simulink model "DroopGFM_sps"  (R2024b)
settings: Solver=ode3  StartTime=0.0  StopTime=10  FixedStep=5e-6  RelTol=1e-3
InitFcn:
  | fsw=10e3;
  | %Ts=1/(fsw*50); %1e-6
  | Ts=1/(fsw*20);  %5e-6
  | 
  | Vodref= 480*sqrt(2/3);
  | Vdc=1000;
  | w0=2*pi*60;
  | 
  | Lf=3.5e-3;
  | Rf=0.1;
  | Cf=50e-6;
  | Lc=0.35e-3;
  | Rc=0.05;
  | 
  | Tci=4/(2*pi*fsw);
  | wci=1/Tci;
  | Kpc=Lf*wci;
  | Kic=Rf*wci;
  | 
  | pm= 50;
  | wcv=1/Tci*(1-sind(pm))/(1+sind(pm));
  | wgc=sqrt(wcv*wci);
  | Kpv=Cf*wgc;
  | Kiv=Kpv*wcv;
  | 
  | mpp = 1.2e-4;
  | 
  | mp1= mpp;
  | mp2= mpp;
  | 
  | nq1=3e-3;
  | nq2=3e-3;
libraries: spsabctodq0Lib x15, slpidlib x12, spsThreePhaseSeriesRLCBranchLib x11, spsThreePhaseVIMeasurementLib x9, spsThreePhaseSeriesRLCLoadLib x4, spsdq0toabcLib x3, spsDCVoltageSourceLib x3, eePowerMeasurement x3, spsGroundLib x3, spsPWMGenerator2LevelLib x3, spsUniversalBridgeLib x3, spsThreePhaseBreakerLib x1
(part 2 of 3)

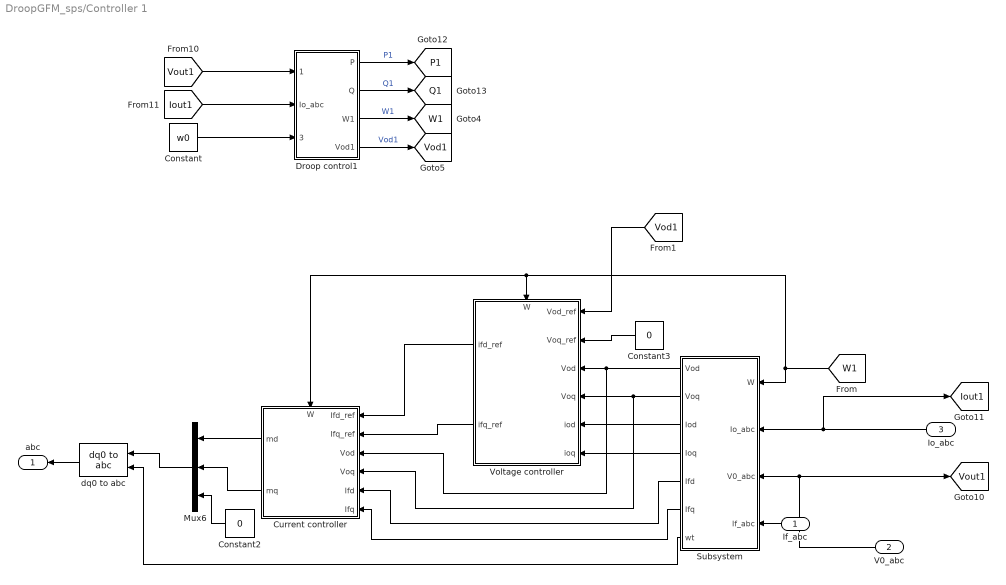
== system DroopGFM_sps/Controller 1 ==
  If_abc : Inport
  V0_abc : Inport  Port=2
  Io_abc : Inport  Port=3
  Constant : Constant  Value=w0
  Constant2 : Constant  Value=0
  Constant3 : Constant  Value=0
  Current controller : Subsystem
      settings: PortSchema="{\"entries\":[{\"content\":{\"sides\":[{\"content\":{\"connectorIds\":[\"In1\",\"In2\",\"In3\",\"In4\",\"In5\",\"In6\"]},\"type\":\"ConnectorPlacement.EquallySpacedRectSide\",\"uuid\":\"afbd0cd8-be12-4bd7-a6dd-f7dac5cf4512\"},{\"content\":{\"connectorIds\":[\"Out1\",\"Out2\"],\"side\":\"RIGHT\"},\"type\":\"ConnectorPlacement.EquallySpacedRectSide\",\"uuid\":\"a2288591-3041-41c1-b291-e9e060e5938f\"},{\"content\":{\"connectorIds\":[\"In7\"],\"side\":\"TOP\"},\"type\":\"ConnectorPlacement.EquallySpacedRectSide\",\"uuid\":\"6bd258a4-7022-4004-b2e3-8400b1f87dc6\"}]},\"type\":\"ConnectorPlacement.EquallySpacedConnector\",\"uuid\":\"ef76f81b-f821-49f2-9550-8127a934c8c3\"}],\"packageUris\":[\"http://schema.mathworks.com/mf0/Connector/R2020b\"],\"version\":\"1.0\"}"
  Droop control1 : Subsystem  SystemSampleTime=0
  Mux6 : Mux  Inputs=3
  Subsystem : Subsystem
  Voltage controller : Subsystem
      settings: PortSchema="{\"entries\":[{\"content\":{\"sides\":[{\"content\":{\"connectorIds\":[\"In1\",\"In2\",\"In3\",\"In4\",\"In5\",\"In6\"]},\"type\":\"ConnectorPlacement.EquallySpacedRectSide\",\"uuid\":\"afbd0cd8-be12-4bd7-a6dd-f7dac5cf4512\"},{\"content\":{\"connectorIds\":[\"Out1\",\"Out2\"],\"side\":\"RIGHT\"},\"type\":\"ConnectorPlacement.EquallySpacedRectSide\",\"uuid\":\"a2288591-3041-41c1-b291-e9e060e5938f\"},{\"content\":{\"connectorIds\":[\"In7\"],\"side\":\"TOP\"},\"type\":\"ConnectorPlacement.EquallySpacedRectSide\",\"uuid\":\"6bd258a4-7022-4004-b2e3-8400b1f87dc6\"}]},\"type\":\"ConnectorPlacement.EquallySpacedConnector\",\"uuid\":\"ef76f81b-f821-49f2-9550-8127a934c8c3\"}],\"packageUris\":[\"http://schema.mathworks.com/mf0/Connector/R2020b\"],\"version\":\"1.0\"}"
  dq0 to abc : spsdq0toabcLib/dq0 to abc  Alignment=90 degrees behind phase A axis
  abc : Outport
  tag scope: Iout1=global, P1=global, Q1=global, Vod1=global, Vout1=global, W1=global
  wires:
  V0_abc/1 -> [Vout1], Subsystem/3(V0_abc)
  Subsystem/5(Ifd) -> Current controller/5(Ifd)
  If_abc/1 -> Subsystem/4(If_abc)
  Voltage controller/1(ifd_ref) -> Current controller/1(Ifd_ref)
  [Vod1] -> Voltage controller/1(Vod_ref)
  [W1] -> Current controller/7(W), Voltage controller/7(W), Subsystem/1(W)
  Current controller/1(md) -> Mux6/1
  Subsystem/4(Ioq) -> Voltage controller/6(ioq)
  Subsystem/7(wt) -> dq0 to abc/2
  Current controller/2(mq) -> Mux6/2
  Io_abc/1 -> [Iout1], Subsystem/2(Io_abc)
  Constant3/1 -> Voltage controller/2(Voq_ref)
  Subsystem/1(Vod) -> Current controller/3(Vod), Voltage controller/3(Vod)
  Mux6/1 -> dq0 to abc/1
  Subsystem/6(Ifq) -> Current controller/6(Ifq)
  Subsystem/3(Iod) -> Voltage controller/5(iod)
  Voltage controller/2(ifq_ref) -> Current controller/2(Ifq_ref)
  Subsystem/2(Voq) -> Current controller/4(Voq), Voltage controller/4(Voq)
  Constant2/1 -> Mux6/3
  dq0 to abc/1 -> abc/1
  Constant/1 -> Droop control1/3(W_nom)
  Droop control1/2(Q) -> [Q1]  "Q1"
  Droop control1/4(Vod1) -> [Vod1]  "Vod1"
  [Vout1] -> Droop control1/1(V0_abc)
  [Iout1] -> Droop control1/2(Io_abc)
  Droop control1/3(W1) -> [W1]  "W1"
  Droop control1/1(P) -> [P1]  "P1"

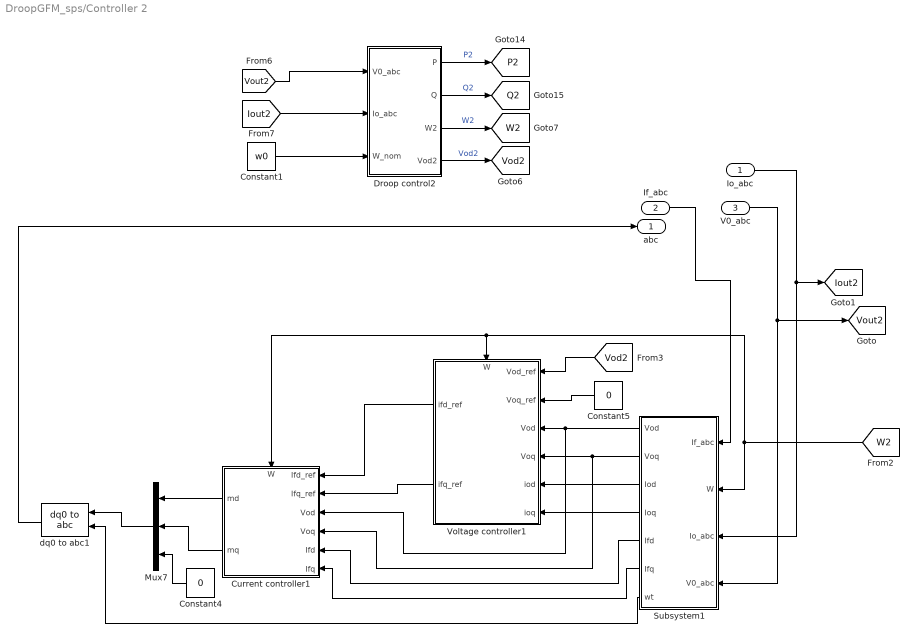
== system DroopGFM_sps/Controller 2 ==
  Io_abc : Inport
  If_abc : Inport  Port=2
  V0_abc : Inport  Port=3
  Constant1 : Constant  Value=w0
  Constant4 : Constant  Value=0
  Constant5 : Constant  Value=0
  Current controller1 : Subsystem
      settings: PortSchema="{\"entries\":[{\"content\":{\"sides\":[{\"content\":{\"connectorIds\":[\"In1\",\"In2\",\"In3\",\"In4\",\"In5\",\"In6\"]},\"type\":\"ConnectorPlacement.EquallySpacedRectSide\",\"uuid\":\"afbd0cd8-be12-4bd7-a6dd-f7dac5cf4512\"},{\"content\":{\"connectorIds\":[\"Out1\",\"Out2\"],\"side\":\"RIGHT\"},\"type\":\"ConnectorPlacement.EquallySpacedRectSide\",\"uuid\":\"a2288591-3041-41c1-b291-e9e060e5938f\"},{\"content\":{\"connectorIds\":[\"In7\"],\"side\":\"TOP\"},\"type\":\"ConnectorPlacement.EquallySpacedRectSide\",\"uuid\":\"6bd258a4-7022-4004-b2e3-8400b1f87dc6\"}]},\"type\":\"ConnectorPlacement.EquallySpacedConnector\",\"uuid\":\"ef76f81b-f821-49f2-9550-8127a934c8c3\"}],\"packageUris\":[\"http://schema.mathworks.com/mf0/Connector/R2020b\"],\"version\":\"1.0\"}"
  Droop control2 : Subsystem
  Mux7 : Mux  Inputs=3
  Subsystem1 : Subsystem
  Voltage controller1 : Subsystem
      settings: PortSchema="{\"entries\":[{\"content\":{\"sides\":[{\"content\":{\"connectorIds\":[\"In1\",\"In2\",\"In3\",\"In4\",\"In5\",\"In6\"]},\"type\":\"ConnectorPlacement.EquallySpacedRectSide\",\"uuid\":\"afbd0cd8-be12-4bd7-a6dd-f7dac5cf4512\"},{\"content\":{\"connectorIds\":[\"Out1\",\"Out2\"],\"side\":\"RIGHT\"},\"type\":\"ConnectorPlacement.EquallySpacedRectSide\",\"uuid\":\"a2288591-3041-41c1-b291-e9e060e5938f\"},{\"content\":{\"connectorIds\":[\"In7\"],\"side\":\"TOP\"},\"type\":\"ConnectorPlacement.EquallySpacedRectSide\",\"uuid\":\"6bd258a4-7022-4004-b2e3-8400b1f87dc6\"}]},\"type\":\"ConnectorPlacement.EquallySpacedConnector\",\"uuid\":\"ef76f81b-f821-49f2-9550-8127a934c8c3\"}],\"packageUris\":[\"http://schema.mathworks.com/mf0/Connector/R2020b\"],\"version\":\"1.0\"}"
  dq0 to abc1 : spsdq0toabcLib/dq0 to abc  Alignment=90 degrees behind phase A axis
  abc : Outport
  tag scope: Iout2=global, P2=global, Q2=global, Vod2=global, Vout2=global, W2=global
  wires:
  [W2] -> Subsystem1/2(W), Current controller1/7(W), Voltage controller1/7(W)
  Constant4/1 -> Mux7/3
  Current controller1/2(mq) -> Mux7/2
  If_abc/1 -> Subsystem1/1(If_abc)
  [Vod2] -> Voltage controller1/1(Vod_ref)
  Subsystem1/4(Ioq) -> Voltage controller1/6(ioq)
  Subsystem1/7(wt) -> dq0 to abc1/2
  dq0 to abc1/1 -> abc/1
  Subsystem1/5(Ifd) -> Current controller1/5(Ifd)
  Mux7/1 -> dq0 to abc1/1
  V0_abc/1 -> [Vout2], Subsystem1/4(V0_abc)
  Voltage controller1/2(ifq_ref) -> Current controller1/2(Ifq_ref)
  Io_abc/1 -> Subsystem1/3(Io_abc), [Iout2]
  Subsystem1/3(Iod) -> Voltage controller1/5(iod)
  Subsystem1/2(Voq) -> Current controller1/4(Voq), Voltage controller1/4(Voq)
  Subsystem1/1(Vod) -> Current controller1/3(Vod), Voltage controller1/3(Vod)
  Constant5/1 -> Voltage controller1/2(Voq_ref)
  Subsystem1/6(Ifq) -> Current controller1/6(Ifq)
  Current controller1/1(md) -> Mux7/1
  Voltage controller1/1(ifd_ref) -> Current controller1/1(Ifd_ref)
  [Iout2] -> Droop control2/2(Io_abc)
  Droop control2/2(Q) -> [Q2]  "Q2"
  Droop control2/1(P) -> [P2]  "P2"
  Droop control2/3(W2) -> [W2]  "W2"
  Droop control2/4(Vod2) -> [Vod2]  "Vod2"
  [Vout2] -> Droop control2/1(V0_abc)
  Constant1/1 -> Droop control2/3(W_nom)

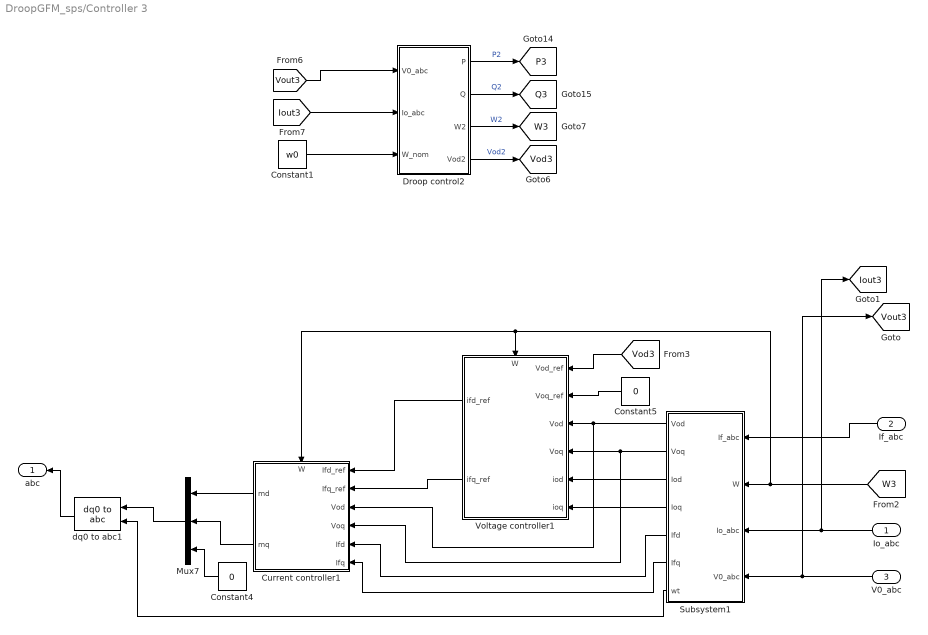
== system DroopGFM_sps/Controller 3 ==
  Io_abc : Inport
  If_abc : Inport  Port=2
  V0_abc : Inport  Port=3
  Constant1 : Constant  Value=w0
  Constant4 : Constant  Value=0
  Constant5 : Constant  Value=0
  Current controller1 : Subsystem
      settings: PortSchema="{\"entries\":[{\"content\":{\"sides\":[{\"content\":{\"connectorIds\":[\"In1\",\"In2\",\"In3\",\"In4\",\"In5\",\"In6\"]},\"type\":\"ConnectorPlacement.EquallySpacedRectSide\",\"uuid\":\"afbd0cd8-be12-4bd7-a6dd-f7dac5cf4512\"},{\"content\":{\"connectorIds\":[\"Out1\",\"Out2\"],\"side\":\"RIGHT\"},\"type\":\"ConnectorPlacement.EquallySpacedRectSide\",\"uuid\":\"a2288591-3041-41c1-b291-e9e060e5938f\"},{\"content\":{\"connectorIds\":[\"In7\"],\"side\":\"TOP\"},\"type\":\"ConnectorPlacement.EquallySpacedRectSide\",\"uuid\":\"6bd258a4-7022-4004-b2e3-8400b1f87dc6\"}]},\"type\":\"ConnectorPlacement.EquallySpacedConnector\",\"uuid\":\"ef76f81b-f821-49f2-9550-8127a934c8c3\"}],\"packageUris\":[\"http://schema.mathworks.com/mf0/Connector/R2020b\"],\"version\":\"1.0\"}"
  Droop control2 : Subsystem
  Mux7 : Mux  Inputs=3
  Subsystem1 : Subsystem
  Voltage controller1 : Subsystem
      settings: PortSchema="{\"entries\":[{\"content\":{\"sides\":[{\"content\":{\"connectorIds\":[\"In1\",\"In2\",\"In3\",\"In4\",\"In5\",\"In6\"]},\"type\":\"ConnectorPlacement.EquallySpacedRectSide\",\"uuid\":\"afbd0cd8-be12-4bd7-a6dd-f7dac5cf4512\"},{\"content\":{\"connectorIds\":[\"Out1\",\"Out2\"],\"side\":\"RIGHT\"},\"type\":\"ConnectorPlacement.EquallySpacedRectSide\",\"uuid\":\"a2288591-3041-41c1-b291-e9e060e5938f\"},{\"content\":{\"connectorIds\":[\"In7\"],\"side\":\"TOP\"},\"type\":\"ConnectorPlacement.EquallySpacedRectSide\",\"uuid\":\"6bd258a4-7022-4004-b2e3-8400b1f87dc6\"}]},\"type\":\"ConnectorPlacement.EquallySpacedConnector\",\"uuid\":\"ef76f81b-f821-49f2-9550-8127a934c8c3\"}],\"packageUris\":[\"http://schema.mathworks.com/mf0/Connector/R2020b\"],\"version\":\"1.0\"}"
  dq0 to abc1 : spsdq0toabcLib/dq0 to abc  Alignment=90 degrees behind phase A axis
  abc : Outport
  tag scope: Iout3=global, P3=global, Q3=global, Vod3=global, Vout3=global, W3=global
  wires:
  Constant1/1 -> Droop control2/3(W_nom)
  [Vout3] -> Droop control2/1(V0_abc)
  Droop control2/4(Vod2) -> [Vod3]  "Vod2"
  Droop control2/3(W2) -> [W3]  "W2"
  Droop control2/1(P) -> [P3]  "P2"
  Droop control2/2(Q) -> [Q3]  "Q2"
  [Iout3] -> Droop control2/2(Io_abc)
  Voltage controller1/1(ifd_ref) -> Current controller1/1(Ifd_ref)
  Current controller1/1(md) -> Mux7/1
  Subsystem1/6(Ifq) -> Current controller1/6(Ifq)
  Constant5/1 -> Voltage controller1/2(Voq_ref)
  Subsystem1/1(Vod) -> Voltage controller1/3(Vod), Current controller1/3(Vod)
  Subsystem1/2(Voq) -> Voltage controller1/4(Voq), Current controller1/4(Voq)
  Subsystem1/3(Iod) -> Voltage controller1/5(iod)
  Io_abc/1 -> [Iout3], Subsystem1/3(Io_abc)
  Voltage controller1/2(ifq_ref) -> Current controller1/2(Ifq_ref)
  V0_abc/1 -> [Vout3], Subsystem1/4(V0_abc)
  Mux7/1 -> dq0 to abc1/1
  Subsystem1/5(Ifd) -> Current controller1/5(Ifd)
  dq0 to abc1/1 -> abc/1
  Subsystem1/7(wt) -> dq0 to abc1/2
  Subsystem1/4(Ioq) -> Voltage controller1/6(ioq)
  [Vod3] -> Voltage controller1/1(Vod_ref)
  If_abc/1 -> Subsystem1/1(If_abc)
  Current controller1/2(mq) -> Mux7/2
  Constant4/1 -> Mux7/3
  [W3] -> Voltage controller1/7(W), Current controller1/7(W), Subsystem1/2(W)

== system DroopGFM_sps/DC source 1 ==
  DC Voltage Source1 : spsDCVoltageSourceLib/DC Voltage Source  Amplitude=Vdc  Measurements=None
  - : PMIOPort  Side=Left
  + : PMIOPort  Port=2  Side=Left
  connections:
  +/RConn1 -- DC Voltage Source1/RConn1
  DC Voltage Source1/LConn1 -- -/RConn1

== system DroopGFM_sps/DC source 2 ==
  DC Voltage Source1 : spsDCVoltageSourceLib/DC Voltage Source  Amplitude=Vdc  Measurements=None
  - : PMIOPort  Side=Left
  + : PMIOPort  Port=2  Side=Left
  connections:
  DC Voltage Source1/LConn1 -- -/RConn1
  +/RConn1 -- DC Voltage Source1/RConn1

== system DroopGFM_sps/DC source 3 ==
  DC Voltage Source1 : spsDCVoltageSourceLib/DC Voltage Source  Amplitude=Vdc  Measurements=None
  - : PMIOPort  Side=Left
  + : PMIOPort  Port=2  Side=Left
  connections:
  +/RConn1 -- DC Voltage Source1/RConn1
  DC Voltage Source1/LConn1 -- -/RConn1

== system DroopGFM_sps/Load 1 ==
  Pload1 : spsThreePhaseVIMeasurementLib/Three-Phase V-I Measurement  VoltageMeasurement=phase-to-ground  SetLabelV=on  LabelV=VL1  Vpu=off  VpuLL=off  CurrentMeasurement=yes  SetLabelI=on  LabelI=IL1  Ipu=off  Pbase=100e6  Vbase=500e3  OutputType=Complex  PhasorSimulation=off  PSBequivalent=0
  Three-Phase Series RLC Load6 : spsThreePhaseSeriesRLCLoadLib/Three-Phase Series RLC Load  LConnTagsString=A|B|C  Configuration=Y (grounded)  NominalVoltage=480  Vabc=[1e3 1e3 1e3]  Vabcp=[1e3 1e3 1e3]  NominalFrequency=60  UnbalancedPower=off  ActivePower=8e3  InductivePower=0.2e3  CapacitivePower=0  Pabc=[10e3 9e3 11e3]  QLabc=[100 90 110]  QCabc=[100 90 110]  Pabcp=[10e3 9e3 11e3]  QLabcp=[100 90 110]  QCabcp=[100 90 110]  Measurements=None  LoadType=constant Z
  A : PMIOPort  Side=Left
  B : PMIOPort  Port=2  Side=Left
  C : PMIOPort  Port=3  Side=Left
  connections:
  Pload1/RConn1 -- Three-Phase Series RLC Load6/LConn1
  Pload1/LConn1 -- A/RConn1
  Pload1/RConn2 -- Three-Phase Series RLC Load6/LConn2
  Pload1/RConn3 -- Three-Phase Series RLC Load6/LConn3
  Pload1/LConn2 -- B/RConn1
  Pload1/LConn3 -- C/RConn1

== system DroopGFM_sps/Load 2 ==
  Pload2 : spsThreePhaseVIMeasurementLib/Three-Phase V-I Measurement  VoltageMeasurement=phase-to-ground  SetLabelV=on  LabelV=VL2  Vpu=off  VpuLL=off  CurrentMeasurement=yes  SetLabelI=on  LabelI=IL2  Ipu=off  Pbase=100e6  Vbase=500e3  OutputType=Complex  PhasorSimulation=off  PSBequivalent=0
  SwL2 : Constant
  Three-Phase Series RLC Load1 : spsThreePhaseSeriesRLCLoadLib/Three-Phase Series RLC Load  LConnTagsString=A|B|C  Configuration=Y (grounded)  NominalVoltage=480  Vabc=[1e3 1e3 1e3]  Vabcp=[1e3 1e3 1e3]  NominalFrequency=60  UnbalancedPower=off  ActivePower=6e3  InductivePower=0.2e3  CapacitivePower=0  Pabc=[10e3 9e3 11e3]  QLabc=[100 90 110]  QCabc=[100 90 110]  Pabcp=[10e3 9e3 11e3]  QLabcp=[100 90 110]  QCabcp=[100 90 110]  Measurements=None  LoadType=constant Z
  Three-Phase Series RLC Load4 : spsThreePhaseSeriesRLCLoadLib/Three-Phase Series RLC Load  LConnTagsString=A|B|C  Configuration=Y (grounded)  NominalVoltage=480  Vabc=[1e3 1e3 1e3]  Vabcp=[1e3 1e3 1e3]  NominalFrequency=60  UnbalancedPower=off  ActivePower=2e3  InductivePower=0  CapacitivePower=0  Pabc=[10e3 9e3 11e3]  QLabc=[100 90 110]  QCabc=[100 90 110]  Pabcp=[10e3 9e3 11e3]  QLabcp=[100 90 110]  QCabcp=[100 90 110]  Measurements=None  LoadType=constant Z
  Three-Phase Breaker : spsThreePhaseBreakerLib/Three-Phase Breaker  InitialState=open  SwitchA=on  SwitchB=on  SwitchC=on  SwitchTimes=[1 2]  External=on  BreakerResistance=0.01  SnubberResistance=1e6  SnubberCapacitance=inf  Measurements=None
  A : PMIOPort  Side=Left
  B : PMIOPort  Port=2  Side=Left
  C : PMIOPort  Port=3  Side=Left
  wires:
  SwL2/1 -> Three-Phase Breaker/1
  connections:
  Three-Phase Series RLC Load1/LConn3 -- Pload2/RConn3 -- Three-Phase Breaker/LConn3
  A/RConn1 -- Pload2/LConn1
  Pload2/LConn3 -- C/RConn1
  Three-Phase Series RLC Load4/LConn1 -- Three-Phase Breaker/RConn1
  Three-Phase Series RLC Load1/LConn2 -- Pload2/RConn2 -- Three-Phase Breaker/LConn2
  Three-Phase Series RLC Load1/LConn1 -- Pload2/RConn1 -- Three-Phase Breaker/LConn1
  Three-Phase Series RLC Load4/LConn2 -- Three-Phase Breaker/RConn2
  Three-Phase Series RLC Load4/LConn3 -- Three-Phase Breaker/RConn3
  Pload2/LConn2 -- B/RConn1

== system DroopGFM_sps/Load 3 ==
  Pload1 : spsThreePhaseVIMeasurementLib/Three-Phase V-I Measurement  VoltageMeasurement=phase-to-ground  SetLabelV=on  LabelV=VL3  Vpu=off  VpuLL=off  CurrentMeasurement=yes  SetLabelI=on  LabelI=IL3  Ipu=off  Pbase=100e6  Vbase=500e3  OutputType=Complex  PhasorSimulation=off  PSBequivalent=0
  Three-Phase Series RLC Load6 : spsThreePhaseSeriesRLCLoadLib/Three-Phase Series RLC Load  LConnTagsString=A|B|C  Configuration=Y (grounded)  NominalVoltage=480  Vabc=[1e3 1e3 1e3]  Vabcp=[1e3 1e3 1e3]  NominalFrequency=60  UnbalancedPower=off  ActivePower=4e3  InductivePower=0.2e3  CapacitivePower=0  Pabc=[10e3 9e3 11e3]  QLabc=[100 90 110]  QCabc=[100 90 110]  Pabcp=[10e3 9e3 11e3]  QLabcp=[100 90 110]  QCabcp=[100 90 110]  Measurements=None  LoadType=constant Z
  A : PMIOPort  Side=Left
  B : PMIOPort  Port=2  Side=Left
  C : PMIOPort  Port=3  Side=Left
  connections:
  Pload1/LConn3 -- C/RConn1
  Pload1/LConn2 -- B/RConn1
  Pload1/RConn3 -- Three-Phase Series RLC Load6/LConn3
  Pload1/RConn2 -- Three-Phase Series RLC Load6/LConn2
  Pload1/LConn1 -- A/RConn1
  Pload1/RConn1 -- Three-Phase Series RLC Load6/LConn1

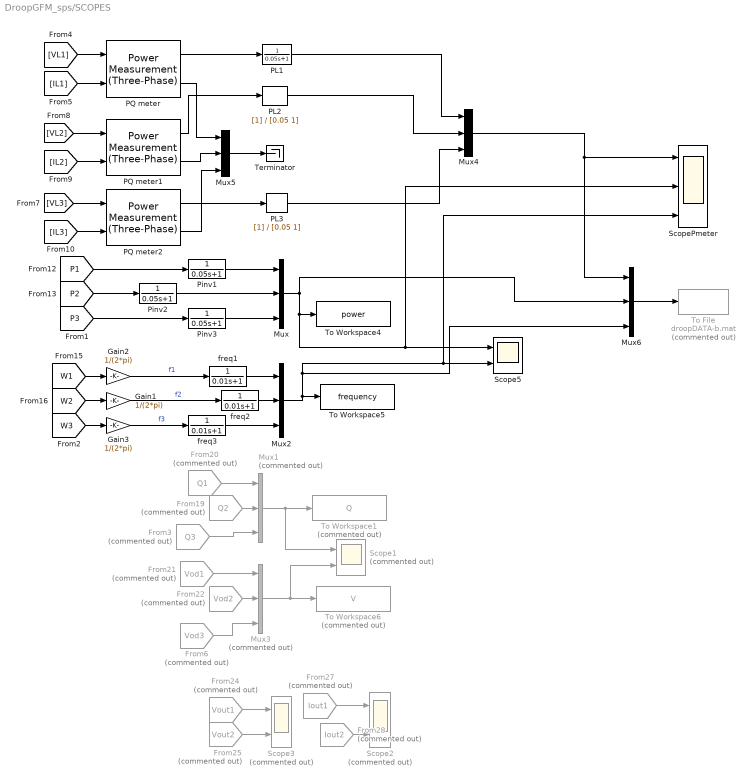
== system DroopGFM_sps/SCOPES ==
  From19 : From  Commented=on  GotoTag=Q2  TagVisibility=global
  From20 : From  Commented=on  GotoTag=Q1  TagVisibility=global
  From21 : From  Commented=on  GotoTag=Vod1  TagVisibility=global
  From22 : From  Commented=on  GotoTag=Vod2  TagVisibility=global
  From24 : From  Commented=on  GotoTag=Vout1  TagVisibility=global
  From25 : From  Commented=on  GotoTag=Vout2  TagVisibility=global
  From27 : From  Commented=on  GotoTag=Iout1  TagVisibility=global
  From28 : From  Commented=on  GotoTag=Iout2  TagVisibility=global
  From3 : From  Commented=on  GotoTag=Q3  TagVisibility=global
  From6 : From  Commented=on  GotoTag=Vod3  TagVisibility=global
  Gain1 : Gain  Gain=1/(2*pi)
  Gain2 : Gain  Gain=1/(2*pi)
  Gain3 : Gain  Gain=1/(2*pi)
  Mux{,2,4..6} (5 alike) : Mux  Inputs=3
  Mux1 : Mux  Commented=on  Inputs=3
  Mux3 : Mux  Commented=on  Inputs=3
  PL1 : TransferFcn  Denominator=[0.05 1]
  PL2 : TransferFcn  Denominator=[0.05 1]
  PL3 : TransferFcn  Denominator=[0.05 1]
  PQ meter : eePowerMeasurement/Power Measurement (Three-Phase)  LabelModeActiveChoice=Discrete  F=60  K=[1]  Seq=Positive  Ts=1e-4
  PQ meter1 : eePowerMeasurement/Power Measurement (Three-Phase)  LabelModeActiveChoice=Discrete  F=60  K=[1]  Seq=Positive  Ts=1e-4
  PQ meter2 : eePowerMeasurement/Power Measurement (Three-Phase)  LabelModeActiveChoice=Discrete  F=60  K=[1]  Seq=Positive  Ts=1e-4
  Pinv1 : TransferFcn  Denominator=[0.05 1]
  Pinv2 : TransferFcn  Denominator=[0.05 1]
  Pinv3 : TransferFcn  Denominator=[0.05 1]
  Scope1 : Scope  Commented=on  NumInputPorts=2
  Scope2 : Scope  Commented=on  NumInputPorts=2
  Scope3 : Scope  Commented=on  NumInputPorts=2
  Scope5 : Scope  NumInputPorts=2
  ScopePmeter : Scope  NumInputPorts=3
  Terminator : Terminator
  To File : ToFile  Commented=on  Filename=droopDATA-b.mat  SaveFormat=Timeseries
  To Workspace1 : ToWorkspace  Commented=on  VariableName=Q  SaveFormat=Structure With Time  SampleTime=-1
  To Workspace4 : ToWorkspace  VariableName=power  SaveFormat=Structure With Time  SampleTime=-1
  To Workspace5 : ToWorkspace  VariableName=frequency  SaveFormat=Structure With Time  SampleTime=-1
  To Workspace6 : ToWorkspace  Commented=on  VariableName=V  SaveFormat=Structure With Time  SampleTime=-1
  freq1 : TransferFcn  Denominator=[0.01 1]
  freq2 : TransferFcn  Denominator=[0.01 1]
  freq3 : TransferFcn  Denominator=[0.01 1]
  wires:
  Mux/1 -> Mux6/2, ScopePmeter/2, Scope5/1, To Workspace4/1
  From20/1 -> Mux1/1
  Mux5/1 -> Terminator/1
  From21/1 -> Mux3/1
  Gain1/1 -> freq2/1  "f2"
  PL2/1 -> Mux4/2
  Mux1/1 -> To Workspace1/1, Scope1/1
  PQ meter/2 -> Mux5/1
  [W1] -> Gain2/1
  From25/1 -> Scope3/2
  [IL1] -> PQ meter/2
  PQ meter1/1 -> PL2/1
  PQ meter1/2 -> Mux5/2
  Gain2/1 -> freq1/1  "f1"
  From22/1 -> Mux3/2
  PQ meter/1 -> PL1/1
  Mux3/1 -> To Workspace6/1, Scope1/2
  Mux4/1 -> Mux6/1, ScopePmeter/1
  From19/1 -> Mux1/2
  [VL2] -> PQ meter1/1
  Mux2/1 -> To Workspace5/1, Mux6/3, ScopePmeter/3, Scope5/2
  [VL1] -> PQ meter/1
  From28/1 -> Scope2/2
  [IL2] -> PQ meter1/2
  PL1/1 -> Mux4/1
  [W2] -> Gain1/1
  From24/1 -> Scope3/1
  From27/1 -> Scope2/1
  [W3] -> Gain3/1
  Gain3/1 -> freq3/1  "f3"
  From3/1 -> Mux1/3
  From6/1 -> Mux3/3
  Mux6/1 -> To File/1
  freq1/1 -> Mux2/1
  freq2/1 -> Mux2/2
  freq3/1 -> Mux2/3
  [P1] -> Pinv1/1
  [P2] -> Pinv2/1
  [P3] -> Pinv3/1
  [IL3] -> PQ meter2/2
  [VL3] -> PQ meter2/1
  PQ meter2/1 -> PL3/1
  PQ meter2/2 -> Mux5/3
  PL3/1 -> Mux4/3
  Pinv1/1 -> Mux/1
  Pinv2/1 -> Mux/2
  Pinv3/1 -> Mux/3

== system DroopGFM_sps/VSC1 ==
  Uref : Inport
  Ground : spsGroundLib/Ground  LConnTagsString=a
  PWM Generator (2-Level) : spsPWMGenerator2LevelLib/PWM Generator (2-Level)  ModulatorType=Three-phase bridge (6 pulses)  ModulatorMode=Unsynchronized  Fc=fsw  Pc=0  nF=27  MinMax="[ -1  1 ]"  SamplingTechnique=Natural  ModulatingSignals=off  m=0.8  Freq=60  Phase=0  Ts=0  ShowCarrierOutport=off
  Three-Phase Series RLC Branch : spsThreePhaseSeriesRLCBranchLib/Three-Phase Series RLC Branch  LConnTagsString=A|B|C  RConnTagsString=A|B|C  BranchType=RL  Resistance=Rf  Inductance=Lf  Capacitance=1e-6  Measurements=None
  Three-Phase Series RLC Branch1 : spsThreePhaseSeriesRLCBranchLib/Three-Phase Series RLC Branch  LConnTagsString=A|B|C  RConnTagsString=A|B|C  BranchType=RL  Resistance=Rc  Inductance=Lc  Capacitance=1e-6  Measurements=None
  Three-Phase Series RLC Branch2 : spsThreePhaseSeriesRLCBranchLib/Three-Phase Series RLC Branch  LConnTagsString=A|B|C  RConnTagsString=A|B|C  BranchType=C  Resistance=1  Inductance=1e-3  Capacitance=Cf  Measurements=None
  Three-Phase V-I Measurement : spsThreePhaseVIMeasurementLib/Three-Phase V-I Measurement  VoltageMeasurement=phase-to-ground  SetLabelV=off  LabelV=Vabc  Vpu=off  VpuLL=off  CurrentMeasurement=yes  SetLabelI=off  LabelI=Iabc  Ipu=off  Pbase=100e6  Vbase=500e3  OutputType=Complex  PhasorSimulation=off  PSBequivalent=0
  Three-Phase V-I Measurement1 : spsThreePhaseVIMeasurementLib/Three-Phase V-I Measurement  VoltageMeasurement=phase-to-ground  SetLabelV=off  LabelV=Vabc  Vpu=off  VpuLL=off  CurrentMeasurement=yes  SetLabelI=off  LabelI=Iabc  Ipu=off  Pbase=100e6  Vbase=500e3  OutputType=Complex  PhasorSimulation=off  PSBequivalent=0
  Universal Bridge : spsUniversalBridgeLib/Universal Bridge  Arms=3  SnubberResistance=1e5  SnubberCapacitance=inf  Device=IGBT / Diodes  Ron=1e-3  Lon=0  ForwardVoltages="[  0  0  ]"  ForwardVoltage=0  GTOparameters=[ 10e-6 , 20e-6 ]  IGBTparameters=[ 1e-6 , 2e-6 ]  Measurements=None  Measurements_2=None  converterType=Rectifier
  P : PMIOPort  Side=Left
  N : PMIOPort  Port=2  Side=Left
  Va : PMIOPort  Port=3  Side=Right
  Vb : PMIOPort  Port=4  Side=Right
  Vc : PMIOPort  Port=5  Side=Right
  Iabc : Outport
  Vabc : Outport  Port=2
  ILf1 : Outport  Port=3
  tag scope: Vt1=global
  wires:
  PWM Generator (2-Level)/1 -> Universal Bridge/1
  Three-Phase V-I Measurement/2 -> Iabc/1
  Three-Phase V-I Measurement/1 -> Vabc/1
  Uref/1 -> PWM Generator (2-Level)/1
  Three-Phase V-I Measurement1/2 -> ILf1/1
  Three-Phase V-I Measurement1/1 -> [Vt1]
  connections:
  Three-Phase Series RLC Branch1/RConn1 -- Va/RConn1
  Three-Phase V-I Measurement1/LConn3 -- Universal Bridge/LConn3
  Three-Phase V-I Measurement/LConn1 -- Three-Phase Series RLC Branch2/LConn1 -- Three-Phase Series RLC Branch/RConn1
  Three-Phase V-I Measurement1/LConn1 -- Universal Bridge/LConn1
  Three-Phase Series RLC Branch/LConn3 -- Three-Phase V-I Measurement1/RConn3
  Three-Phase V-I Measurement1/LConn2 -- Universal Bridge/LConn2
  Three-Phase Series RLC Branch1/RConn3 -- Vc/RConn1
  Three-Phase Series RLC Branch/LConn1 -- Three-Phase V-I Measurement1/RConn1
  Vb/RConn1 -- Three-Phase Series RLC Branch1/RConn2
  Three-Phase V-I Measurement/RConn3 -- Three-Phase Series RLC Branch1/LConn3
  Three-Phase Series RLC Branch/LConn2 -- Three-Phase V-I Measurement1/RConn2
  Three-Phase V-I Measurement/RConn1 -- Three-Phase Series RLC Branch1/LConn1
  Three-Phase V-I Measurement/LConn3 -- Three-Phase Series RLC Branch2/LConn3 -- Three-Phase Series RLC Branch/RConn3
  Three-Phase V-I Measurement/LConn2 -- Three-Phase Series RLC Branch2/LConn2 -- Three-Phase Series RLC Branch/RConn2
  Three-Phase V-I Measurement/RConn2 -- Three-Phase Series RLC Branch1/LConn2
  Three-Phase Series RLC Branch2/RConn3 -- Three-Phase Series RLC Branch2/RConn1 -- Three-Phase Series RLC Branch2/RConn2 -- Ground/LConn1
  P/RConn1 -- Universal Bridge/RConn1
  N/RConn1 -- Universal Bridge/RConn2

== system DroopGFM_sps/VSC2 ==
  Uref : Inport
  Ground : spsGroundLib/Ground  LConnTagsString=a
  PWM Generator (2-Level) : spsPWMGenerator2LevelLib/PWM Generator (2-Level)  ModulatorType=Three-phase bridge (6 pulses)  ModulatorMode=Unsynchronized  Fc=fsw  Pc=0  nF=27  MinMax="[ -1  1 ]"  SamplingTechnique=Natural  ModulatingSignals=off  m=0.8  Freq=60  Phase=0  Ts=0  ShowCarrierOutport=off
  Three-Phase Series RLC Branch : spsThreePhaseSeriesRLCBranchLib/Three-Phase Series RLC Branch  LConnTagsString=A|B|C  RConnTagsString=A|B|C  BranchType=RL  Resistance=Rf  Inductance=Lf  Capacitance=1e-6  Measurements=None
  Three-Phase Series RLC Branch1 : spsThreePhaseSeriesRLCBranchLib/Three-Phase Series RLC Branch  LConnTagsString=A|B|C  RConnTagsString=A|B|C  BranchType=RL  Resistance=Rc  Inductance=Lc  Capacitance=1e-6  Measurements=None
  Three-Phase Series RLC Branch2 : spsThreePhaseSeriesRLCBranchLib/Three-Phase Series RLC Branch  LConnTagsString=A|B|C  RConnTagsString=A|B|C  BranchType=C  Resistance=1  Inductance=1e-3  Capacitance=Cf  Measurements=None
  Three-Phase V-I Measurement : spsThreePhaseVIMeasurementLib/Three-Phase V-I Measurement  VoltageMeasurement=phase-to-ground  SetLabelV=off  LabelV=Vabc  Vpu=off  VpuLL=off  CurrentMeasurement=yes  SetLabelI=off  LabelI=Iabc  Ipu=off  Pbase=100e6  Vbase=500e3  OutputType=Complex  PhasorSimulation=off  PSBequivalent=0
  Three-Phase V-I Measurement1 : spsThreePhaseVIMeasurementLib/Three-Phase V-I Measurement  VoltageMeasurement=phase-to-ground  SetLabelV=off  LabelV=Vabc  Vpu=off  VpuLL=off  CurrentMeasurement=yes  SetLabelI=off  LabelI=Iabc  Ipu=off  Pbase=100e6  Vbase=500e3  OutputType=Complex  PhasorSimulation=off  PSBequivalent=0
  Universal Bridge : spsUniversalBridgeLib/Universal Bridge  Arms=3  SnubberResistance=1e5  SnubberCapacitance=inf  Device=IGBT / Diodes  Ron=1e-3  Lon=0  ForwardVoltages="[  0  0  ]"  ForwardVoltage=0  GTOparameters=[ 10e-6 , 20e-6 ]  IGBTparameters=[ 1e-6 , 2e-6 ]  Measurements=None  Measurements_2=None  converterType=Rectifier
  N : PMIOPort  Side=Left
  P : PMIOPort  Port=2  Side=Left
  Vc : PMIOPort  Port=3  Side=Right
  Vb : PMIOPort  Port=4  Side=Right
  Va : PMIOPort  Port=5  Side=Right
  Vabc : Outport
  ILf1 : Outport  Port=2
  Iabc : Outport  Port=3
  tag scope: Vt2=global
  wires:
  Three-Phase V-I Measurement1/1 -> [Vt2]
  Three-Phase V-I Measurement1/2 -> ILf1/1
  Uref/1 -> PWM Generator (2-Level)/1
  Three-Phase V-I Measurement/1 -> Vabc/1
  Three-Phase V-I Measurement/2 -> Iabc/1
  PWM Generator (2-Level)/1 -> Universal Bridge/1
  connections:
  N/RConn1 -- Universal Bridge/RConn2
  P/RConn1 -- Universal Bridge/RConn1
  Ground/LConn1 -- Three-Phase Series RLC Branch2/RConn2 -- Three-Phase Series RLC Branch2/RConn1 -- Three-Phase Series RLC Branch2/RConn3
  Three-Phase V-I Measurement/RConn2 -- Three-Phase Series RLC Branch1/LConn2
  Three-Phase Series RLC Branch/RConn2 -- Three-Phase Series RLC Branch2/LConn2 -- Three-Phase V-I Measurement/LConn2
  Three-Phase Series RLC Branch/RConn3 -- Three-Phase Series RLC Branch2/LConn3 -- Three-Phase V-I Measurement/LConn3
  Three-Phase V-I Measurement/RConn1 -- Three-Phase Series RLC Branch1/LConn1
  Three-Phase Series RLC Branch/LConn2 -- Three-Phase V-I Measurement1/RConn2
  Three-Phase V-I Measurement/RConn3 -- Three-Phase Series RLC Branch1/LConn3
  Vb/RConn1 -- Three-Phase Series RLC Branch1/RConn2
  Three-Phase Series RLC Branch/LConn1 -- Three-Phase V-I Measurement1/RConn1
  Three-Phase Series RLC Branch1/RConn3 -- Vc/RConn1
  Three-Phase V-I Measurement1/LConn2 -- Universal Bridge/LConn2
  Three-Phase Series RLC Branch/LConn3 -- Three-Phase V-I Measurement1/RConn3
  Three-Phase V-I Measurement1/LConn1 -- Universal Bridge/LConn1
  Three-Phase Series RLC Branch/RConn1 -- Three-Phase Series RLC Branch2/LConn1 -- Three-Phase V-I Measurement/LConn1
  Three-Phase V-I Measurement1/LConn3 -- Universal Bridge/LConn3
  Three-Phase Series RLC Branch1/RConn1 -- Va/RConn1

== system DroopGFM_sps/VSC3 ==
  Uref : Inport
  Ground : spsGroundLib/Ground  LConnTagsString=a
  PWM Generator (2-Level) : spsPWMGenerator2LevelLib/PWM Generator (2-Level)  ModulatorType=Three-phase bridge (6 pulses)  ModulatorMode=Unsynchronized  Fc=fsw  Pc=0  nF=27  MinMax="[ -1  1 ]"  SamplingTechnique=Natural  ModulatingSignals=off  m=0.8  Freq=60  Phase=0  Ts=0  ShowCarrierOutport=off
  Three-Phase Series RLC Branch : spsThreePhaseSeriesRLCBranchLib/Three-Phase Series RLC Branch  LConnTagsString=A|B|C  RConnTagsString=A|B|C  BranchType=RL  Resistance=Rf  Inductance=Lf  Capacitance=1e-6  Measurements=None
  Three-Phase Series RLC Branch1 : spsThreePhaseSeriesRLCBranchLib/Three-Phase Series RLC Branch  LConnTagsString=A|B|C  RConnTagsString=A|B|C  BranchType=RL  Resistance=Rc  Inductance=Lc  Capacitance=1e-6  Measurements=None
  Three-Phase Series RLC Branch2 : spsThreePhaseSeriesRLCBranchLib/Three-Phase Series RLC Branch  LConnTagsString=A|B|C  RConnTagsString=A|B|C  BranchType=C  Resistance=1  Inductance=1e-3  Capacitance=Cf  Measurements=None
  Three-Phase V-I Measurement : spsThreePhaseVIMeasurementLib/Three-Phase V-I Measurement  VoltageMeasurement=phase-to-ground  SetLabelV=off  LabelV=Vabc  Vpu=off  VpuLL=off  CurrentMeasurement=yes  SetLabelI=off  LabelI=Iabc  Ipu=off  Pbase=100e6  Vbase=500e3  OutputType=Complex  PhasorSimulation=off  PSBequivalent=0
  Three-Phase V-I Measurement1 : spsThreePhaseVIMeasurementLib/Three-Phase V-I Measurement  VoltageMeasurement=phase-to-ground  SetLabelV=off  LabelV=Vabc  Vpu=off  VpuLL=off  CurrentMeasurement=yes  SetLabelI=off  LabelI=Iabc  Ipu=off  Pbase=100e6  Vbase=500e3  OutputType=Complex  PhasorSimulation=off  PSBequivalent=0
  Universal Bridge : spsUniversalBridgeLib/Universal Bridge  Arms=3  SnubberResistance=1e5  SnubberCapacitance=inf  Device=IGBT / Diodes  Ron=1e-3  Lon=0  ForwardVoltages="[  0  0  ]"  ForwardVoltage=0  GTOparameters=[ 10e-6 , 20e-6 ]  IGBTparameters=[ 1e-6 , 2e-6 ]  Measurements=None  Measurements_2=None  converterType=Rectifier
  N : PMIOPort  Side=Left
  P : PMIOPort  Port=2  Side=Left
  Vc : PMIOPort  Port=3  Side=Right
  Vb : PMIOPort  Port=4  Side=Right
  Va : PMIOPort  Port=5  Side=Right
  Vabc : Outport
  ILf1 : Outport  Port=2
  Iabc : Outport  Port=3
  tag scope: Vt3=global
  wires:
  PWM Generator (2-Level)/1 -> Universal Bridge/1
  Three-Phase V-I Measurement/2 -> Iabc/1
  Three-Phase V-I Measurement/1 -> Vabc/1
  Uref/1 -> PWM Generator (2-Level)/1
  Three-Phase V-I Measurement1/2 -> ILf1/1
  Three-Phase V-I Measurement1/1 -> [Vt3]
  connections:
  Three-Phase Series RLC Branch1/RConn1 -- Va/RConn1
  Three-Phase V-I Measurement1/LConn3 -- Universal Bridge/LConn3
  Three-Phase V-I Measurement/LConn1 -- Three-Phase Series RLC Branch2/LConn1 -- Three-Phase Series RLC Branch/RConn1
  Three-Phase V-I Measurement1/LConn1 -- Universal Bridge/LConn1
  Three-Phase Series RLC Branch/LConn3 -- Three-Phase V-I Measurement1/RConn3
  Three-Phase V-I Measurement1/LConn2 -- Universal Bridge/LConn2
  Three-Phase Series RLC Branch1/RConn3 -- Vc/RConn1
  Three-Phase Series RLC Branch/LConn1 -- Three-Phase V-I Measurement1/RConn1
  Vb/RConn1 -- Three-Phase Series RLC Branch1/RConn2
  Three-Phase V-I Measurement/RConn3 -- Three-Phase Series RLC Branch1/LConn3
  Three-Phase Series RLC Branch/LConn2 -- Three-Phase V-I Measurement1/RConn2
  Three-Phase V-I Measurement/RConn1 -- Three-Phase Series RLC Branch1/LConn1
  Three-Phase V-I Measurement/LConn3 -- Three-Phase Series RLC Branch2/LConn3 -- Three-Phase Series RLC Branch/RConn3
  Three-Phase V-I Measurement/LConn2 -- Three-Phase Series RLC Branch2/LConn2 -- Three-Phase Series RLC Branch/RConn2
  Three-Phase V-I Measurement/RConn2 -- Three-Phase Series RLC Branch1/LConn2
  Three-Phase Series RLC Branch2/RConn3 -- Three-Phase Series RLC Branch2/RConn1 -- Three-Phase Series RLC Branch2/RConn2 -- Ground/LConn1
  P/RConn1 -- Universal Bridge/RConn1
  N/RConn1 -- Universal Bridge/RConn2

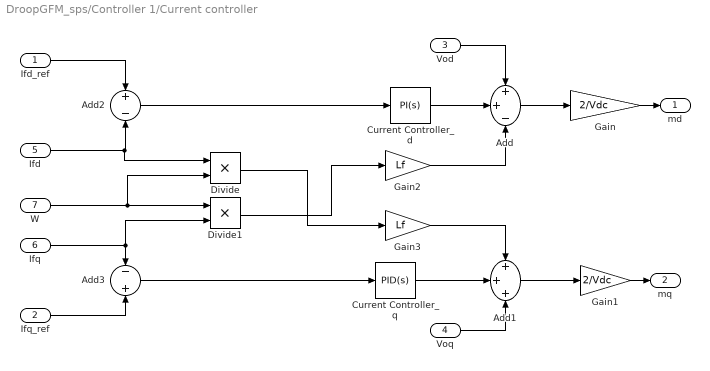
== system DroopGFM_sps/Controller 1/Current controller ==
  Ifd_ref : Inport
  Ifq_ref : Inport  Port=2
  Vod : Inport  Port=3
  Voq : Inport  Port=4
  Ifd : Inport  Port=5
  Ifq : Inport  Port=6
  W : Inport  Port=7
  Add : Sum  Inputs=++-
  Add1 : Sum  Inputs=+++
  Add2 : Sum  Inputs=+-
  Add3 : Sum  Inputs=-+
  Current Controller_d : slpidlib/PID Controller  Controller=PI  Form=Parallel  TimeDomain=Continuous-time  UseExternalTs=off  SampleTime=-1  IntegratorMethod=Forward Euler  FilterMethod=Forward Euler  ControllerParametersSource=internal  P=Kpc  I=Kic  UseKiTs=off  D=0  UseExternalDerivativeSource=off  N=100  UseFilter=on  TunerSelectOption=Transfer Function Based (PID Tuner App)  InitialConditionSource=internal  InitialConditionForIntegrator=0  InitialConditionForFilter=0  DifferentiatorICPrevScaledInput=0  ExternalReset=none  TrackingMode=off  Kt=1  LimitOutput=off  SatLimitsSource=internal  UpperSaturationLimit=inf  LowerSaturationLimit=-inf  LinearizeAsGain=on  AntiWindupMode=none  Kb=1  LimitIntegrator=off  UpperIntegratorSaturationLimit=inf  LowerIntegratorSaturationLimit=-inf  POutMin=[]  POutMax=[]  IOutMin=[]  IOutMax=[]  DOutMin=[]  DOutMax=[]  NOutMin=[]  NOutMax=[]  SumOutMin=[]  SumOutMax=[]  SaturationOutMin=[]  SaturationOutMax=[]  PParamMin=[]  PParamMax=[]  IParamMin=[]  IParamMax=[]  DParamMin=[]  DParamMax=[]  NParamMin=[]  NParamMax=[]  KbParamMin=[]  KbParamMax=[]  KtParamMin=[]  KtParamMax=[]  KbOutMin=[]  KbOutMax=[]  KtOutMin=[]  KtOutMax=[]  IntegratorOutMin=[]  IntegratorOutMax=[]  FilterOutMin=[]  FilterOutMax=[]  SumI1OutMin=[]  SumI1OutMax=[]  SumI2OutMin=[]  SumI2OutMax=[]  SumI3OutMin=[]  SumI3OutMax=[]  SumI4OutMin=[]  SumI4OutMax=[]  SumDOutMin=[]  SumDOutMax=[]  DifferentiatorOutMin=[]  DifferentiatorOutMax=[]  FilterDiffOutCoefMin=[]  FilterDiffOutCoefMax=[]  ReciprocalOutMin=[]  ReciprocalOutMax=[]  SumDenOutMin=[]  SumDenOutMax=[]  SumNumOutMin=[]  SumNumOutMax=[]  DivideOutMin=[]  DivideOutMax=[]  UdiffTsProdOutMin=[]  UdiffTsProdOutMax=[]  NTsProdOutMin=[]  NTsProdOutMax=[]  UintegralTsProdOutMin=[]  UintegralTsProdOutMax=[]  UngainTsProdOutMin=[]  UngainTsProdOutMax=[]  ClampingZeroOutDataTypeStr=Inherit: Inherit via back propagation  ClampingZeroOutMin=[]  ClampingZeroOutMax=[]  FilterDenConstantOutDataTypeStr=Inherit: Inherit via back propagation  FilterDenConstantOutMin=[]  FilterDenConstantOutMax=[]  PCopyOutDataTypeStr=Inherit: Inherit via back propagation  PCopyOutMin=[]  PCopyOutMax=[]  NCopyOutDataTypeStr=Inherit: Inherit via back propagation  NCopyOutMin=[]  NCopyOutMax=[]  IntegratorContinuousStateAttributes=''  IntegratorStateMustResolveToSignalObject=off  IntegratorRTWStateStorageClass=Auto  FilterContinuousStateAttributes=''  FilterStateMustResolveToSignalObject=off  FilterRTWStateStorageClass=Auto  ParallelPVariant=InternalParameters  IdealPVariant=Disabled  IVariant=InternalParameters  DVariant=Disabled  IntegratorVariant=Continuous  SatVariant=Disabled  AWVariant=Passthrough  PCopyVariant=Disabled  TRVariant=Disabled  FdbkBlocksVariant=Forward  IdealPFdbkVariant=Disabled  SatFdbkVariant=Disabled  DerivativeFilterVariant=Disabled  NVariant=Disabled  NCopyVariant=Disabled_SignalSpec  FilterICVariant=Disabled  IntegratorICVariant=InternalICs  ExternalResetVariant=Disabled  TRSumVariant=Passthrough  SumFdbkVariant=Disabled  SumVariant=Sum_PI  TsampFilterVariant=InternalTs  TsampNgainVariant=Passthrough  TsampIntegralVariant=Disabled_SignalSpec  ExternalSaturationOutDataTypeStr=Inherit: Same as second input  DerivativeSourceVariant=Disabled  PreIntVariant=InternalPreInt
  Current Controller_q : slpidlib/PID Controller  Controller=PID  Form=Parallel  TimeDomain=Continuous-time  UseExternalTs=off  SampleTime=-1  IntegratorMethod=Forward Euler  FilterMethod=Forward Euler  ControllerParametersSource=internal  P=Kpc  I=Kic  UseKiTs=off  D=0  UseExternalDerivativeSource=off  N=100  UseFilter=on  TunerSelectOption=Transfer Function Based (PID Tuner App)  InitialConditionSource=internal  InitialConditionForIntegrator=0  InitialConditionForFilter=0  DifferentiatorICPrevScaledInput=0  ExternalReset=none  TrackingMode=off  Kt=1  LimitOutput=off  SatLimitsSource=internal  UpperSaturationLimit=inf  LowerSaturationLimit=-inf  LinearizeAsGain=on  AntiWindupMode=none  Kb=1  LimitIntegrator=off  UpperIntegratorSaturationLimit=inf  LowerIntegratorSaturationLimit=-inf  POutMin=[]  POutMax=[]  IOutMin=[]  IOutMax=[]  DOutMin=[]  DOutMax=[]  NOutMin=[]  NOutMax=[]  SumOutMin=[]  SumOutMax=[]  SaturationOutMin=[]  SaturationOutMax=[]  PParamMin=[]  PParamMax=[]  IParamMin=[]  IParamMax=[]  DParamMin=[]  DParamMax=[]  NParamMin=[]  NParamMax=[]  KbParamMin=[]  KbParamMax=[]  KtParamMin=[]  KtParamMax=[]  KbOutMin=[]  KbOutMax=[]  KtOutMin=[]  KtOutMax=[]  IntegratorOutMin=[]  IntegratorOutMax=[]  FilterOutMin=[]  FilterOutMax=[]  SumI1OutMin=[]  SumI1OutMax=[]  SumI2OutMin=[]  SumI2OutMax=[]  SumI3OutMin=[]  SumI3OutMax=[]  SumI4OutMin=[]  SumI4OutMax=[]  SumDOutMin=[]  SumDOutMax=[]  DifferentiatorOutMin=[]  DifferentiatorOutMax=[]  FilterDiffOutCoefMin=[]  FilterDiffOutCoefMax=[]  ReciprocalOutMin=[]  ReciprocalOutMax=[]  SumDenOutMin=[]  SumDenOutMax=[]  SumNumOutMin=[]  SumNumOutMax=[]  DivideOutMin=[]  DivideOutMax=[]  UdiffTsProdOutMin=[]  UdiffTsProdOutMax=[]  NTsProdOutMin=[]  NTsProdOutMax=[]  UintegralTsProdOutMin=[]  UintegralTsProdOutMax=[]  UngainTsProdOutMin=[]  UngainTsProdOutMax=[]  ClampingZeroOutDataTypeStr=Inherit: Inherit via back propagation  ClampingZeroOutMin=[]  ClampingZeroOutMax=[]  FilterDenConstantOutDataTypeStr=Inherit: Inherit via back propagation  FilterDenConstantOutMin=[]  FilterDenConstantOutMax=[]  PCopyOutDataTypeStr=Inherit: Inherit via back propagation  PCopyOutMin=[]  PCopyOutMax=[]  NCopyOutDataTypeStr=Inherit: Inherit via back propagation  NCopyOutMin=[]  NCopyOutMax=[]  IntegratorContinuousStateAttributes=''  IntegratorStateMustResolveToSignalObject=off  IntegratorRTWStateStorageClass=Auto  FilterContinuousStateAttributes=''  FilterStateMustResolveToSignalObject=off  FilterRTWStateStorageClass=Auto  ParallelPVariant=InternalParameters  IdealPVariant=Disabled  IVariant=InternalParameters  DVariant=InternalParameters  IntegratorVariant=Continuous  SatVariant=Disabled  AWVariant=Passthrough  PCopyVariant=Disabled  TRVariant=Disabled  FdbkBlocksVariant=Forward  IdealPFdbkVariant=Disabled  SatFdbkVariant=Disabled  DerivativeFilterVariant=ContFilter  NVariant=InternalParameters  NCopyVariant=Disabled  FilterICVariant=InternalICsFilter  IntegratorICVariant=InternalICs  ExternalResetVariant=Disabled  TRSumVariant=Passthrough  SumFdbkVariant=Disabled  SumVariant=Sum_PID  TsampFilterVariant=InternalTs  TsampNgainVariant=Passthrough  TsampIntegralVariant=Disabled_SignalSpec  ExternalSaturationOutDataTypeStr=Inherit: Same as second input  DerivativeSourceVariant=ErrorSignal  PreIntVariant=InternalPreInt
  Divide : Product  Inputs=**
  Divide1 : Product  Inputs=**
  Gain : Gain  Gain=2/Vdc
  Gain1 : Gain  Gain=2/Vdc
  Gain2 : Gain  Gain=Lf
  Gain3 : Gain  Gain=Lf
  md : Outport
  mq : Outport  Port=2
  wires:
  Voq/1 -> Add1/3
  Ifd_ref/1 -> Add2/1
  Ifq_ref/1 -> Add3/2
  Gain3/1 -> Add1/1
  Current Controller_q/1 -> Add1/2
  Gain2/1 -> Add/3
  Vod/1 -> Add/1
  Add/1 -> Gain/1
  Add2/1 -> Current Controller_d/1
  Add3/1 -> Current Controller_q/1
  Add1/1 -> Gain1/1
  Current Controller_d/1 -> Add/2
  Gain1/1 -> mq/1
  Gain/1 -> md/1
  Ifd/1 -> Divide/1, Add2/2
  Divide/1 -> Gain3/1
  W/1 -> Divide1/1, Divide/2
  Divide1/1 -> Gain2/1
  Ifq/1 -> Add3/1, Divide1/2

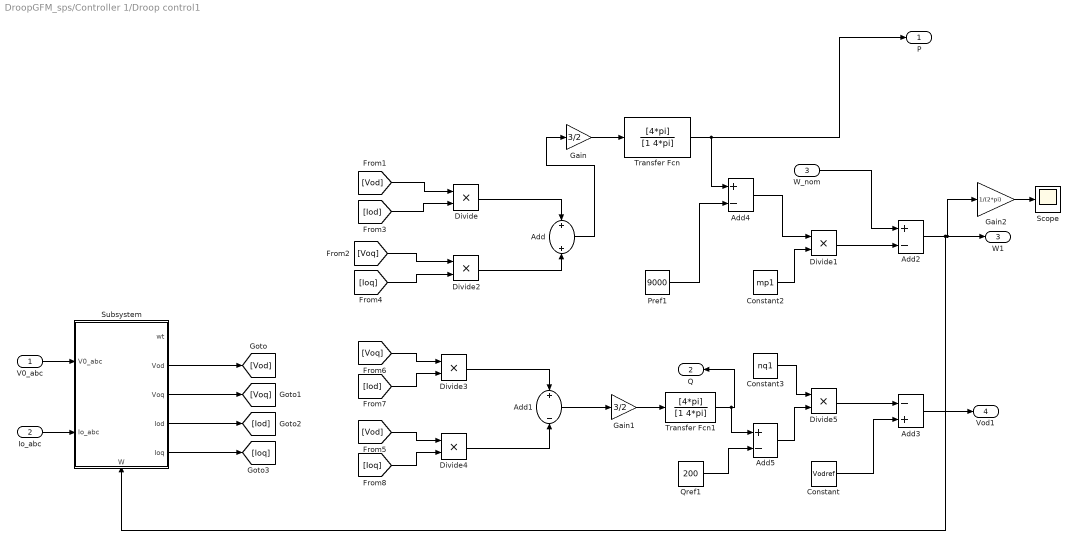
== system DroopGFM_sps/Controller 1/Droop control1 ==
  V0_abc : Inport
  Io_abc : Inport  Port=2
  W_nom : Inport  Port=3
  Add : Sum
  Add{1..2,4..5} (4 alike) : Sum  Inputs=+-
  Add3 : Sum  Inputs=-+
  Constant : Constant  Value=Vodref
  Constant2 : Constant  Value=mp1
  Constant3 : Constant  Value=nq1
  Divide{,1..5} (6 alike) : Product  Inputs=**
  Gain : Gain  Gain=3/2
  Gain1 : Gain  Gain=3/2
  Gain2 : Gain  Gain=1/(2*pi)
  Pref1 : Constant  Value=9000
  Qref1 : Constant  Value=200
  Scope : Scope
  Subsystem : Subsystem
      settings: PortSchema="{\"entries\":[{\"content\":{\"sides\":[{\"content\":{\"connectorIds\":[\"In1\",\"In2\"]},\"type\":\"ConnectorPlacement.EquallySpacedRectSide\",\"uuid\":\"3c0ce44c-1409-4df9-aab1-2e1a82b43481\"},{\"content\":{\"connectorIds\":[\"Out1\",\"Out2\",\"Out3\",\"Out4\",\"Out5\"],\"side\":\"RIGHT\"},\"type\":\"ConnectorPlacement.EquallySpacedRectSide\",\"uuid\":\"4a9336a4-679f-4f93-987c-a9f8549bd21c\"},{\"content\":{\"connectorIds\":[],\"side\":\"TOP\"},\"type\":\"ConnectorPlacement.EquallySpacedRectSide\",\"uuid\":\"6340f487-ff74-466e-845e-7d1050881641\"},{\"content\":{\"connectorIds\":[\"In3\"],\"side\":\"BOTTOM\"},\"type\":\"ConnectorPlacement.EquallySpacedRectSide\",\"uuid\":\"1e1d92d0-8955-434a-9fbd-76af504505ea\"}]},\"type\":\"ConnectorPlacement.EquallySpacedConnector\",\"uuid\":\"bfddd833-a64a-4f18-a4bd-88042aac52a3\"}],\"packageUris\":[\"http://schema.mathworks.com/mf0/Connector/R2020b\"],\"version\":\"1.0\"}"
  Transfer Fcn : TransferFcn  Numerator=[4*pi]  Denominator=[1 4*pi]  ParameterTunability=Optimized
  Transfer Fcn1 : TransferFcn  Numerator=[4*pi]  Denominator=[1 4*pi]  ParameterTunability=Optimized
  P : Outport
  Q : Outport  Port=2
  W1 : Outport  Port=3
  Vod1 : Outport  Port=4
  wires:
  Subsystem/2(Vod) -> [Vod]
  Subsystem/3(Voq) -> [Voq]
  Subsystem/4(Iod) -> [Iod]
  Subsystem/5(Ioq) -> [Ioq]
  [Vod] -> Divide/1
  [Iod] -> Divide/2
  [Voq] -> Divide2/1
  [Ioq] -> Divide2/2
  Divide/1 -> Add/1
  Divide2/1 -> Add/2
  Add/1 -> Gain/1
  [Voq] -> Divide3/1
  [Iod] -> Divide3/2
  [Vod] -> Divide4/1
  [Ioq] -> Divide4/2
  Divide3/1 -> Add1/1
  Divide4/1 -> Add1/2
  Add1/1 -> Gain1/1
  W_nom/1 -> Add2/1
  Divide1/1 -> Add2/2
  Divide5/1 -> Add3/1
  Constant/1 -> Add3/2
  Constant2/1 -> Divide1/2
  Constant3/1 -> Divide5/1
  Add2/1 -> Gain2/1, W1/1, Subsystem/3(W)
  Add3/1 -> Vod1/1
  Gain/1 -> Transfer Fcn/1
  Transfer Fcn/1 -> Add4/1, P/1
  Gain1/1 -> Transfer Fcn1/1
  Transfer Fcn1/1 -> Add5/1, Q/1
  Io_abc/1 -> Subsystem/2(Io_abc)
  V0_abc/1 -> Subsystem/1(V0_abc)
  Gain2/1 -> Scope/1
  Add4/1 -> Divide1/1
  Pref1/1 -> Add4/2
  Qref1/1 -> Add5/2
  Add5/1 -> Divide5/2

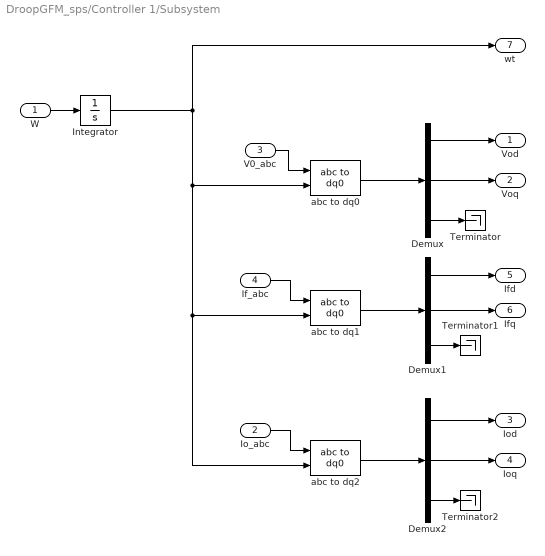
== system DroopGFM_sps/Controller 1/Subsystem ==
  W : Inport
  Io_abc : Inport  Port=2
  V0_abc : Inport  Port=3
  If_abc : Inport  Port=4
  Demux : Demux  Outputs=3
  Demux1 : Demux  Outputs=3
  Demux2 : Demux  Outputs=3
  Integrator : Integrator
  Terminator : Terminator
  Terminator1 : Terminator
  Terminator2 : Terminator
  abc to dq0 : spsabctodq0Lib/abc to dq0  Alignment=90 degrees behind phase A axis
  abc to dq1 : spsabctodq0Lib/abc to dq0  Alignment=90 degrees behind phase A axis
  abc to dq2 : spsabctodq0Lib/abc to dq0  Alignment=90 degrees behind phase A axis
  Vod : Outport
  Voq : Outport  Port=2
  Iod : Outport  Port=3
  Ioq : Outport  Port=4
  Ifd : Outport  Port=5
  Ifq : Outport  Port=6
  wt : Outport  Port=7
  wires:
  Demux2/3 -> Terminator2/1
  Demux/3 -> Terminator/1
  abc to dq0/1 -> Demux/1
  Demux2/2 -> Ioq/1
  Demux2/1 -> Iod/1
  abc to dq1/1 -> Demux1/1
  Demux1/2 -> Ifq/1
  Demux1/1 -> Ifd/1
  abc to dq2/1 -> Demux2/1
  Demux1/3 -> Terminator1/1
  If_abc/1 -> abc to dq1/1
  Integrator/1 -> abc to dq2/2, abc to dq1/2, abc to dq0/2, wt/1
  V0_abc/1 -> abc to dq0/1
  Io_abc/1 -> abc to dq2/1
  W/1 -> Integrator/1
  Demux/2 -> Voq/1
  Demux/1 -> Vod/1
